simulink library "bpm_dq_S_noH_D_RL_U_HA_Spin_xk"  (R2022b)
settings: Solver=VariableStepAuto  StartTime=0.0  StopTime=10.0  RelTol=1e-3
Description:
  | Created by MapleSim.
settings Model: Creator=MapleSim  LastModifiedBy=BEDNASA

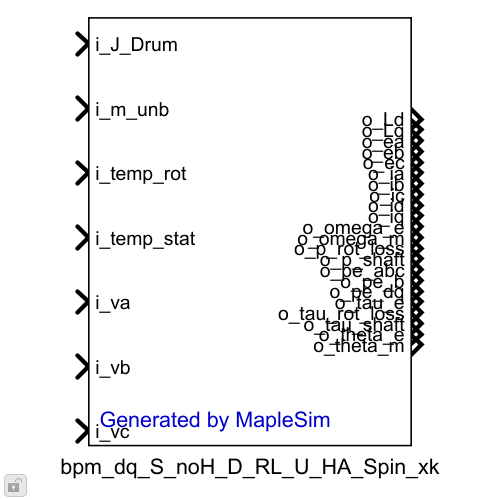
[thumbnail: Simulink's stored preview of the top-level diagram]
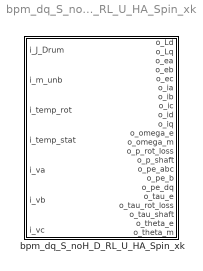
== system bpm_dq_S_noH_D_RL_U_HA_Spin_xk ==
  bpm_dq_S_noH_D_RL_U_HA_Spin_xk : Subsystem  Description=Subsystem: bpm_dq_S_noH_D_RL_U_HA_Spin_xk  mask(bpm_dq_S_noH_D_RL_U_HA_Spin_xk){ic=[0., 0., 0., -0., 0.], Par1=.1e-3, Par2=0., Par3=1., Par4=2., Par5=3., Par6=4., Par7=5., Par8=6., Par9=7., Par10=.515e-3, Par11=.884e-1, Par12=.2117e-1, Par13=.2117e-1, Par14=.2117e-1, Par15=.2117e-1, Par16=.2117e-1, Par17=.2117e-1, Par18=.2117e-1, Par19=.2117e-1, Par20=.972e-1, Par21=.2744e-1, Par22=.2777e-1, Par23=.2742e-1, Par24=.2646e-1, Par25=.2426e-1, Par26=.2329e-1, Par27=.2241e-1, Par28=.2241e-1, Par29=1., Par30=3., Par31=0., Par32=1., Par33=12., Par34=19., Par35=26., Par36=35., Par37=41., Par38=56., Par39=0., Par40=.5e3, Par41=.3e4, Par42=.4e4, Par43=.5e4, Par44=.7e4, Par45=.12e5, Par46=.18e5, Par47=1., Par48=.1e2, Par49=9.15, Par50=1., Par51=2., Par52=3., Par53=22., Par54=22., Par55=.2e-3, Par56=.4e-2, Par57=.206e-2, Par58=.1151, Par59=1., Par60=1., Par61=1., Par62=0., Par63=0., Par64=0., Par65=-9.8, Par66=-1., Par67=1., ExtData=, MinStep=1/40, TimeStep_Solver=1e-4}
      mask prompts: ic "Initial Conditions:"; Par1 "SHDRLUHAS1_B:"; Par2 "SHDRLUHAS1_I_pk0:"; Par3 "SHDRLUHAS1_I_pk1:"; Par4 "SHDRLUHAS1_I_pk2:"; Par5 "SHDRLUHAS1_I_pk3:"; Par6 "SHDRLUHAS1_I_pk4:"; Par7 "SHDRLUHAS1_I_pk5:"; Par8 "SHDRLUHAS1_I_pk6:"; Par9 "SHDRLUHAS1_I_pk7:"; Par10 "SHDRLUHAS1_Jrotor:"; Par11 "SHDRLUHAS1_Ld0:"; Par12 "SHDRLUHAS1_Ld_a0:"; Par13 "SHDRLUHAS1_Ld_a1:"; Par14 "SHDRLUHAS1_Ld_a2:"; Par15 "SHDRLUHAS1_Ld_a3:"; Par16 "SHDRLUHAS1_Ld_a4:"; Par17 "SHDRLUHAS1_Ld_a5:"; Par18 "SHDRLUHAS1_Ld_a6:"; Par19 "SHDRLUHAS1_Ld_a7:"; Par20 "SHDRLUHAS1_Lq0:"; Par21 "SHDRLUHAS1_Lq_b0:"; Par22 "SHDRLUHAS1_Lq_b1:"; Par23 "SHDRLUHAS1_Lq_b2:"; Par24 "SHDRLUHAS1_Lq_b3:"; Par25 "SHDRLUHAS1_Lq_b4:"; Par26 "SHDRLUHAS1_Lq_b5:"; Par27 "SHDRLUHAS1_Lq_b6:"; Par28 "SHDRLUHAS1_Lq_b7:"; Par29 "SHDRLUHAS1_Ls_Sat_enable:"; Par30 "SHDRLUHAS1_NPP:"; Par31 "SHDRLUHAS1_Rot_Loss_Power0:"; Par32 "SHDRLUHAS1_Rot_Loss_Power1:"; Par33 "SHDRLUHAS1_Rot_Loss_Power2:"; Par34 "SHDRLUHAS1_Rot_Loss_Power3:"; Par35 "SHDRLUHAS1_Rot_Loss_Power4:"; Par36 "SHDRLUHAS1_Rot_Loss_Power5:"; Par37 "SHDRLUHAS1_Rot_Loss_Power6:"; Par38 "SHDRLUHAS1_Rot_Loss_Power7:"; Par39 "SHDRLUHAS1_Rot_Loss_Speed0:"; Par40 "SHDRLUHAS1_Rot_Loss_Speed1:"; Par41 "SHDRLUHAS1_Rot_Loss_Speed2:"; Par42 "SHDRLUHAS1_Rot_Loss_Speed3:"; Par43 "SHDRLUHAS1_Rot_Loss_Speed4:"; Par44 "SHDRLUHAS1_Rot_Loss_Speed5:"; Par45 "SHDRLUHAS1_Rot_Loss_Speed6:"; Par46 "SHDRLUHAS1_Rot_Loss_Speed7:"; Par47 "SHDRLUHAS1_Rot_Loss_enable:"; Par48 "SHDRLUHAS1_Rot_Loss_omega_th:"; Par49 "SHDRLUHAS1_Rs0:"; Par50 "SHDRLUHAS1_Rsa_aux:"; Par51 "SHDRLUHAS1_Rsb_aux:"; Par52 "SHDRLUHAS1_Rsc_aux:"; Par53 "SHDRLUHAS1_TrRef:"; Par54 "SHDRLUHAS1_TsRef:"; Par55 "SHDRLUHAS1_Ts:"; Par56 "SHDRLUHAS1_alpha_s:"; Par57 "SHDRLUHAS1_d_magnet:"; Par58 "SHDRLUHAS1_phiPM1:"; Par59 "SHDRLUHAS1_HA_Spin_Mechanics_CF:"; Par60 "SHDRLUHAS1_HA_Spin_Mechanics_TR:"; Par61 "SHDRLUHAS1_HA_Spin_Mechanics_damp:"; Par62 "SHDRLUHAS1_HA_Spin_Mechanics_damper3_1_B:"; Par63 "SHDRLUHAS1_HA_Spin_Mechanics_damper3_1_C:"; Par64 "SHDRLUHAS1_HA_Spin_Mechanics_fixed_phi0:"; Par65 "SHDRLUHAS1_HA_Spin_Mechanics_gain11_k:"; Par66 "SHDRLUHAS1_HA_Spin_Mechanics_gain21_k:"; Par67 "SHDRLUHAS1_HA_Spin_Mechanics_r_unb:"; ExtData "Extended Visualization Data - File Name (leave blank to disable):"; MinStep "Extended Visualization Data - Minimum Sample Step:"; TimeStep_Solver "Time Step - Solver:"
      mask help:
      | Variable Definitions
      |
      | Variable(s) in the Initial Condition Vector:
      |      x[ 0] = `Main.SHDRLUHAS1.o_id`(t)
      |      x[ 1] = `Main.SHDRLUHAS1.o_iq`(t)
      |      x[ 2] = `Main.SHDRLUHAS1.o_omega_e`(t)
      |      x[ 3] = `Main.SHDRLUHAS1.o_theta_e`(t)
      |      x[ 4] = diff(`Main.SHDRLUHAS1.o_theta_e`(t),t)
      |
      | Variable(s) in the Output Vector:
      |    o_Ld:
      |      y[ 0] = `Main.SHDRLUHAS1.o_Ld`(t)
      |    o_Lq:
      |      y[ 1] = `Main.SHDRLUHAS1.o_Lq`(t)
      |    o_ea:
      |      y[ 2] = `Main.SHDRLUHAS1.o_ea`(t)
      |    o_eb:
      |      y[ 3] = `Main.SHDRLUHAS1.o_eb`(t)
      |    o_ec:
      |      y[ 4] = `Main.SHDRLUHAS1.o_ec`(t)
      |    o_ia:
      |      y[ 5] = `Main.SHDRLUHAS1.o_ia`(t)
      |    o_ib:
      |      y[ 6] = `Main.SHDRLUHAS1.o_ib`(t)
      |    o_ic:
      |      y[ 7] = `Main.SHDRLUHAS1.o_ic`(t)
      |    o_id:
      |      y[ 8] = `Main.SHDRLUHAS1.o_id`(t)
      |    o_iq:
      |      y[ 9] = `Main.SHDRLUHAS1.o_iq`(t)
      |    o_omega_e:
      |      y[10] = `Main.SHDRLUHAS1.o_omega_e`(t)
      |    o_omega_m:
      |      y[11] = `Main.SHDRLUHAS1.o_omega_m`(t)
      |    o_p_rot_loss:
      |      y[12] = `Main.SHDRLUHAS1.o_p_rot_loss`(t)
      |    o_p_shaft:
      |      y[13] = `Main.SHDRLUHAS1.o_p_shaft`(t)
      |    o_pe_abc:
      |      y[14] = `Main.SHDRLUHAS1.o_pe_abc`(t)
      |    o_pe_b:
      |      y[15] = `Main.SHDRLUHAS1.o_pe_b`(t)
      |    o_pe_dq:
      |      y[16] = `Main.SHDRLUHAS1.o_pe_dq`(t)
      |    o_tau_e:
      |      y[17] = `Main.SHDRLUHAS1.o_tau_e`(t)
      |    o_tau_rot_loss:
      |      y[18] = `Main.SHDRLUHAS1.o_tau_rot_loss`(t)
      |    o_tau_shaft:
      |      y[19] = `Main.SHDRLUHAS1.o_tau_shaft`(t)
      |    o_theta_e:
      |      y[20] = `Main.SHDRLUHAS1.o_theta_e`(t)
      |    o_theta_m:
      |      y[21] = `Main.SHDRLUHAS1.o_theta_m`(t)
      |
      | Variable(s) in the Input Vector:
      |    i_J_Drum:
      |      y[ 0] = `Main.SHDRLUHAS1.i_J_Drum`(t)
      |    i_m_unb:
      |      y[ 1] = `Main.SHDRLUHAS1.i_m_unb`(t)
      |    i_temp_rot:
      |      y[ 2] = `Main.SHDRLUHAS1.i_temp_rot`(t)
      |    i_temp_stat:
      |      y[ 3] = `Main.SHDRLUHAS1.i_temp_stat`(t)
      |    i_va:
      |      y[ 4] = `Main.SHDRLUHAS1.i_va`(t)
      |    i_vb:
      |      y[ 5] = `Main.SHDRLUHAS1.i_vb`(t)
      |    i_vc:
      |      y[ 6] = `Main.SHDRLUHAS1.i_vc`(t)
      |
      | Parameter(s):
      |      p[ 0] = `Main.SHDRLUHAS1.B` (default = .1e-3)
      |      p[ 1] = `Main.SHDRLUHAS1.I_pk0` (default = 0.)
      |      p[ 2] = `Main.SHDRLUHAS1.I_pk1` (default = 1.)
      |      p[ 3] = `Main.SHDRLUHAS1.I_pk2` (default = 2.)
      |      p[ 4] = `Main.SHDRLUHAS1.I_pk3` (default = 3.)
      |      p[ 5] = `Main.SHDRLUHAS1.I_pk4` (default = 4.)
      |      p[ 6] = `Main.SHDRLUHAS1.I_pk5` (default = 5.)
      |      p[ 7] = `Main.SHDRLUHAS1.I_pk6` (default = 6.)
      |      p[ 8] = `Main.SHDRLUHAS1.I_pk7` (default = 7.)
      |      p[ 9] = `Main.SHDRLUHAS1.Jrotor` (default = .515e-3)
      |      p[10] = `Main.SHDRLUHAS1.Ld0` (default = .884e-1)
      |      p[11] = `Main.SHDRLUHAS1.Ld_a0` (default = .2117e-1)
      |      p[12] = `Main.SHDRLUHAS1.Ld_a1` (default = .2117e-1)
      |      p[13] = `Main.SHDRLUHAS1.Ld_a2` (default = .2117e-1)
      |      p[14] = `Main.SHDRLUHAS1.Ld_a3` (default = .2117e-1)
      |      p[15] = `Main.SHDRLUHAS1.Ld_a4` (default = .2117e-1)
      |      p[16] = `Main.SHDRLUHAS1.Ld_a5` (default = .2117e-1)
      |      p[17] = `Main.SHDRLUHAS1.Ld_a6` (default = .2117e-1)
      |      p[18] = `Main.SHDRLUHAS1.Ld_a7` (default = .2117e-1)
      |      p[19] = `Main.SHDRLUHAS1.Lq0` (default = .972e-1)
      |      p[20] = `Main.SHDRLUHAS1.Lq_b0` (default = .2744e-1)
      |      p[21] = `Main.SHDRLUHAS1.Lq_b1` (default = .2777e-1)
      |      p[22] = `Main.SHDRLUHAS1.Lq_b2` (default = .2742e-1)
      |      p[23] = `Main.SHDRLUHAS1.Lq_b3` (default = .2646e-1)
      |      p[24] = `Main.SHDRLUHAS1.Lq_b4` (default = .2426e-1)
      |      p[25] = `Main.SHDRLUHAS1.Lq_b5` (default = .2329e-1)
      |      p[26] = `Main.SHDRLUHAS1.Lq_b6` (default = .2241e-1)
      |      p[27] = `Main.SHDRLUHAS1.Lq_b7` (default = .2241e-1)
      |      p[28] = `Main.SHDRLUHAS1.Ls_Sat_enable` (default = 1.)
      |      p[29] = `Main.SHDRLUHAS1.NPP` (default = 3.)
      |      p[30] = `Main.SHDRLUHAS1.Rot_Loss_Power0` (default = 0.)
      |      p[31] = `Main.SHDRLUHAS1.Rot_Loss_Power1` (default = 1.)
      |      p[32] = `Main.SHDRLUHAS1.Rot_Loss_Power2` (default = 12.)
      |      p[33] = `Main.SHDRLUHAS1.Rot_Loss_Power3` (default = 19.)
      |      p[34] = `Main.SHDRLUHAS1.Rot_Loss_Power4` (default = 26.)
      |      p[35] = `Main.SHDRLUHAS1.Rot_Loss_Power5` (default = 35.)
      |      p[36] = `Main.SHDRLUHAS1.Rot_Loss_Power6` (default = 41.)
      |      p[37] = `Main.SHDRLUHAS1.Rot_Loss_Power7` (default = 56.)
      |      p[38] = `Main.SHDRLUHAS1.Rot_Loss_Speed0` (default = 0.)
      |      p[39] = `Main.SHDRLUHAS1.Rot_Loss_Speed1` (default = .5e3)
      |      p[40] = `Main.SHDRLUHAS1.Rot_Loss_Speed2` (default = .3e4)
      |      p[41] = `Main.SHDRLUHAS1.Rot_Loss_Speed3` (default = .4e4)
      |      p[42] = `Main.SHDRLUHAS1.Rot_Loss_Speed4` (default = .5e4)
      |      p[43] = `Main.SHDRLUHAS1.Rot_Loss_Speed5` (default = .7e4)
      |      p[44] = `Main.SHDRLUHAS1.Rot_Loss_Speed6` (default = .12e5)
      |      p[45] = `Main.SHDRLUHAS1.Rot_Loss_Speed7` (default = .18e5)
      |      p[46] = `Main.SHDRLUHAS1.Rot_Loss_enable` (default = 1.)
      |      p[47] = `Main.SHDRLUHAS1.Rot_Loss_omega_th` (default = .1e2)
      |      p[48] = `Main.SHDRLUHAS1.Rs0` (default = 9.15)
      |      p[49] = `Main.SHDRLUHAS1.Rsa_aux` (default = 1.)
      |      p[50] = `Main.SHDRLUHAS1.Rsb_aux` (default = 2.)
      |      p[51] = `Main.SHDRLUHAS1.Rsc_aux` (default = 3.)
      |      p[52] = `Main.SHDRLUHAS1.TrRef` (default = 22.)
      |      p[53] = `Main.SHDRLUHAS1.TsRef` (default = 22.)
      |      p[54] = `Main.SHDRLUHAS1.Ts` (default = .2e-3)
      |      p[55] = `Main.SHDRLUHAS1.alpha_s` (default = .4e-2)
      |      p[56] = `Main.SHDRLUHAS1.d_magnet` (default = .206e-2)
      |      p[57] = `Main.SHDRLUHAS1.phiPM1` (default = .1151)
      |      p[58] = `Main.SHDRLUHAS1.HA_Spin_Mechanics.CF` (default = 1.)
      |      p[59] = `Main.SHDRLUHAS1.HA_Spin_Mechanics.TR` (default = 1.)
      |      p[60] = `Main.SHDRLUHAS1.HA_Spin_Mechanics.damp` (default = 1.)
      |      p[61] = `Main.SHDRLUHAS1.HA_Spin_Mechanics.damper3_1.B` (default = 0.)
      |      p[62] = `Main.SHDRLUHAS1.HA_Spin_Mechanics.damper3_1.C` (default = 0.)
      |      p[63] = `Main.SHDRLUHAS1.HA_Spin_Mechanics.fixed.phi0` (default = 0.)
      |      p[64] = `Main.SHDRLUHAS1.HA_Spin_Mechanics.gain11.k` (default = -9.8)
      |      p[65] = `Main.SHDRLUHAS1.HA_Spin_Mechanics.gain21.k` (default = -1.)
      |      p[66] = `Main.SHDRLUHAS1.HA_Spin_Mechanics.r_unb` (default = 1.)
      mask Help: <!DOCTYPE html PUBLIC "-//W3C//DTD HTML 4.01 Transitional//EN" "http://www.w3.org/TR/1999/REC-html401-19991224/loose.dtd"> <html lang="en"> <head> <title>bpm_dq_S_noH_D_RL_U_HA_Spin_xk :: MapleSim model</title> <style type="text/css"> body { background-color: white; margin:10px;} h1 { color: #990000; font-size: x-large; } h2 { color: #990000; font-size: large; margin-top:0ex;     margin-bottom:0ex;   font-weight:bold;  } h3 { color:#990000;  margin-top:0ex;   margin-bottom:0ex;  font-weight:bold;    font-size: medium; } h4 { color:black;    margin-top:0ex;   margin-bottom:0ex;  font-weight:bold;    font-size: medium; } /* Vertical space in tables other than the header and footer banners */ table.body { margin-top: 2ex; margin-bottom: 2ex;} /* Make the text shrink to fit narrow windows, but not stretch too far in wide windows. */ p,h1,h2,div.content div { max-width: 600px; } pre.codeinput { background: #EEEEEE; padding: 10px;} @media print { pre.codeinput { word-wrap:break-word; width:100%; } } span.keyword { color: #0000FF} span.comment { color: #228B22} span.string { color: #A020F0} span.untermstring {color: #B20000} span.syscmd { color: #B28C00} pre.error { color: red;} p.footer { text-align: right; font-size: xx-small; font-weight: lighter; font-style: italic; color: gray; } </style> <meta name="generator" content="DocBook XSL Stylesheets V1.52.2"> <meta name="chunktype" content="refpage"> <meta http-equiv="Content-Script-Type" content="text/javascript"> </head> <body> <a name="top_of_page"></a> <p style="font-size:1px;"> <a name="f8-894621"></a> <a name="transferfcn"></a> <a class="indexterm" name="zmw57dd0e42758"></a></p> <h1 class="reftitle">bpm_dq_S_noH_D_RL_U_HA_Spin_xk</h1> <p>Simulink Block generated by MapleSim Connector</p> <p><a name="f8-894627"></a></p> <h1>Description <span class="inlinemediaobject"></span></h1> <p><a class="indexterm" name="zmw57dd0e42781"></a></p> <p>The bpm_dq_S_noH_D_RL_U_HA_Spin_xk model runs in the continuous domain and is created in the MapleSim modeling environment. The discrete S-Function block bpm_dq_S_noH_D_RL_U_HA_Spin_xk is created using MapleSim Connector. The block is a 7-input, 22-output, 67-parameter system.</p> <p><a name="f8-894641"></a></p> <h1>System Variables</h1> <p>The following variables are used in the S-Function block:</p>  State Variable(s)<dl><dd>x[ 0] = `Main.SHDRLUHAS1.o_id`(t)</dd></br><dd>x[ 1] = `Main.SHDRLUHAS1.o_iq`(t)</dd></br><dd>x[ 2] = `Main.SHDRLUHAS1.o_omega_e`(t)</dd></br><dd>x[ 3] = `Main.SHDRLUHAS1.o_theta_e`(t)</dd></br><dd>x[ 4] = diff(`Main.SHDRLUHAS1.o_theta_e`(t),t)</dd></br></dl> Output Variable(s)<dl><dd>o_Ld:</dd></br><dd>&nbsp;&nbsp;y[ 0] = `Main.SHDRLUHAS1.o_Ld`(t)</dd></br><dd>o_Lq:</dd></br><dd>&nbsp;&nbsp;y[ 1] = `Main.SHDRLUHAS1.o_Lq`(t)</dd></br><dd>o_ea:</dd></br><dd>&nbsp;&nbsp;y[ 2] = `Main.SHDRLUHAS1.o_ea`(t)</dd></br><dd>o_eb:</dd></br><dd>&nbsp;&nbsp;y[ 3] = `Main.SHDRLUHAS1.o_eb`(t)</dd></br><dd>o_ec:</dd></br><dd>&nbsp;&nbsp;y[ 4] = `Main.SHDRLUHAS1.o_ec`(t)</dd></br><dd>o_ia:</dd></br><dd>&nbsp;&nbsp;y[ 5] = `Main.SHDRLUHAS1.o_ia`(t)</dd></br><dd>o_ib:</dd></br><dd>&nbsp;&nbsp;y[ 6] = `Main.SHDRLUHAS1.o_ib`(t)</dd></br><dd>o_ic:</dd></br><dd>&nbsp;&nbsp;y[ 7] = `Main.SHDRLUHAS1.o_ic`(t)</dd></br><dd>o_id:</dd></br><dd>&nbsp;&nbsp;y[ 8] = `Main.SHDRLUHAS1.o_id`(t)</dd></br><dd>o_iq:</dd></br><dd>&nbsp;&nbsp;y[ 9] = `Main.SHDRLUHAS1.o_iq`(t)</dd></br><dd>o_omega_e:</dd></br><dd>&nbsp;&nbsp;y[10] = `Main.SHDRLUHAS1.o_omega_e`(t)</dd></br><dd>o_omega_m:</dd></br><dd>&nbsp;&nbsp;y[11] = `Main.SHDRLUHAS1.o_omega_m`(t)</dd></br><dd>o_p_rot_loss:</dd></br><dd>&nbsp;&nbsp;y[12] = `Main.SHDRLUHAS1.o_p_rot_loss`(t)</dd></br><dd>o_p_shaft:</dd></br><dd>&nbsp;&nbsp;y[13] = `Main.SHDRLUHAS1.o_p_shaft`(t)</dd></br><dd>o_pe_abc:</dd></br><dd>&nbsp;&nbsp;y[14] = `Main.SHDRLUHAS1.o_pe_abc`(t)</dd></br><dd>o_pe_b:</dd></br><dd>&nbsp;&nbsp;y[15] = `Main.SHDRLUHAS1.o_pe_b`(t)</dd></br><dd>o_pe_dq:</dd></br><dd>&nbsp;&nbsp;y[16] = `Main.SHDRLUHAS1.o_pe_dq`(t)</dd></br><dd>o_tau_e:</dd></br><dd>&nbsp;&nbsp;y[17] = `Main.SHDRLUHAS1.o_tau_e`(t)</dd></br><dd>o_tau_rot_loss:</dd></br><dd>&nbsp;&nbsp;y[18] = `Main.SHDRLUHAS1.o_tau_rot_loss`(t)</dd></br><dd>o_tau_shaft:</dd></br><dd>&nbsp;&nbsp;y[19] = `Main.SHDRLUHAS1.o_tau_shaft`(t)</dd></br><dd>o_theta_e:</dd></br><dd>&nbsp;&nbsp;y[20] = `Main.SHDRLUHAS1.o_theta_e`(t)</dd></br><dd>o_theta_m:</dd></br><dd>&nbsp;&nbsp;y[21] = `Main.SHDRLUHAS1.o_theta_m`(t)</dd></br></dl> Input Variable(s)<dl><dd>i_J_Drum:</dd></br><dd>&nbsp;&nbsp;y[ 0] = `Main.SHDRLUHAS1.i_J_Drum`(t)</dd></br><dd>i_m_unb:</dd></br><dd>&nbsp;&nbsp;y[ 1] = `Main.SHDRLUHAS1.i_m_unb`(t)</dd></br><dd>i_temp_rot:</dd></br><dd>&nbsp;&nbsp;y[ 2] = `Main.SHDRLUHAS1.i_temp_rot`(t)</dd></br><dd>i_temp_stat:</dd></br><dd>&nbsp;&nbsp;y[ 3] = `Main.SHDRLUHAS1.i_temp_stat`(t)</dd></br><dd>i_va:</dd></br><dd>&nbsp;&nbsp;y[ 4] = `Main.SHDRLUHAS1.i_va`(t)</dd></br><dd>i_vb:</dd></br><dd>&nbsp;&nbsp;y[ 5] = `Main.SHDRLUHAS1.i_vb`(t)</dd></br><dd>i_vc:</dd></br><dd>&nbsp;&nbsp;y[ 6] = `Main.SHDRLUHAS1.i_vc`(t)</dd></br></dl> Parameter(s)<dl><dd>p[ 0] = `Main.SHDRLUHAS1.B` (default = .1e-3)</dd></br><dd>p[ 1] = `Main.SHDRLUHAS1.I_pk0` (default = 0.)</dd></br><dd>p[ 2] = `Main.SHDRLUHAS1.I_pk1` (default = 1.)</dd></br><dd>p[ 3] = `Main.SHDRLUHAS1.I_pk2` (default = 2.)</dd></br><dd>p[ 4] = `Main.SHDRLUHAS1.I_pk3` (default = 3.)</dd></br><dd>p[ 5] = `Main.SHDRLUHAS1.I_pk4` (default = 4.)</dd></br><dd>p[ 6] = `Main.SHDRLUHAS1.I_pk5` (default = 5.)</dd></br><dd>p[ 7] = `Main.SHDRLUHAS1.I_pk6` (default = 6.)</dd></br><dd>p[ 8] = `Main.SHDRLUHAS1.I_pk7` (default = 7.)</dd></br><dd>p[ 9] = `Main.SHDRLUHAS1.Jrotor` (default = .515e-3)</dd></br><dd>p[10] = `Main.SHDRLUHAS1.Ld0` (default = .884e-1)</dd></br><dd>p[11] = `Main.SHDRLUHAS1.Ld_a0` (default = .2117e-1)</dd></br><dd>p[12] = `Main.SHDRLUHAS1.Ld_a1` (default = .2117e-1)</dd></br><dd>p[13] = `Main.SHDRLUHAS1.Ld_a2` (default = .2117e-1)</dd></br><dd>p[14] = `Main.SHDRLUHAS1.Ld_a3` (default = .2117e-1)</dd></br><dd>p[15] = `Main.SHDRLUHAS1.Ld_a4` (default = .2117e-1)</dd></br><dd>p[16] = `Main.SHDRLUHAS1.Ld_a5` (default = .2117e-1)</dd></br><dd>p[17] = `Main.SHDRLUHAS1.Ld_a6` (default = .2117e-1)</dd></br><dd>p[18] = `Main.SHDRLUHAS1.Ld_a7` (default = .2117e-1)</dd></br><dd>p[19] = `Main.SHDRLUHAS1.Lq0` (default = .972e-1)</dd></br><dd>p[20] = `Main.SHDRLUHAS1.Lq_b0` (default = .2744e-1)</dd></br><dd>p[21] = `Main.SHDRLUHAS1.Lq_b1` (default = .2777e-1)</dd></br><dd>p[22] = `Main.SHDRLUHAS1.Lq_b2` (default = .2742e-1)</dd></br><dd>p[23] = `Main.SHDRLUHAS1.Lq_b3` (default = .2646e-1)</dd></br><dd>p[24] = `Main.SHDRLUHAS1.Lq_b4` (default = .2426e-1)</dd></br><dd>p[25] = `Main.SHDRLUHAS1.Lq_b5` (default = .2329e-1)</dd></br><dd>p[26] = `Main.SHDRLUHAS1.Lq_b6` (default = .2241e-1)</dd></br><dd>p[27] = `Main.SHDRLUHAS1.Lq_b7` (default = .2241e-1)</dd></br><dd>p[28] = `Main.SHDRLUHAS1.Ls_Sat_enable` (default = 1.)</dd></br><dd>p[29] = `Main.SHDRLUHAS1.NPP` (default = 3.)</dd></br><dd>p[30] = `Main.SHDRLUHAS1.Rot_Loss_Power0` (default = 0.)</dd></br><dd>p[31] = `Main.SHDRLUHAS1.Rot_Loss_Power1` (default = 1.)</dd></br><dd>p[32] = `Main.SHDRLUHAS1.Rot_Loss_Power2` (default = 12.)</dd></br><dd>p[33] = `Main.SHDRLUHAS1.Rot_Loss_Power3` (default = 19.)</dd></br><dd>p[34] = `Main.SHDRLUHAS1.Rot_Loss_Power4` (default = 26.)</dd></br><dd>p[35] = `Main.SHDRLUHAS1.Rot_Loss_Power5` (default = 35.)</dd></br><dd>p[36] = `Main.SHDRLUHAS1.Rot_Loss_Power6` (default = 41.)</dd></br><dd>p[37] = `Main.SHDRLUHAS1.Rot_Loss_Power7` (default = 56.)</dd></br><dd>p[38] = `Main.SHDRLUHAS1.Rot_Loss_Speed0` (default = 0.)</dd></br><dd>p[39] = `Main.SHDRLUHAS1.Rot_Loss_Speed1` (default = .5e3)</dd></br><dd>p[40] = `Main.SHDRLUHAS1.Rot_Loss_Speed2` (default = .3e4)</dd></br><dd>p[41] = `Main.SHDRLUHAS1.Rot_Loss_Speed3` (default = .4e4)</dd></br><dd>p[42] = `Main.SHDRLUHAS1.Rot_Loss_Speed4` (default = .5e4)</dd></br><dd>p[43] = `Main.SHDRLUHAS1.Rot_Loss_Speed5` (default = .7e4)</dd></br><dd>p[44] = `Main.SHDRLUHAS1.Rot_Loss_Speed6` (default = .12e5)</dd></br><dd>p[45] = `Main.SHDRLUHAS1.Rot_Loss_Speed7` (default = .18e5)</dd></br><dd>p[46] = `Main.SHDRLUHAS1.Rot_Loss_enable` (default = 1.)</dd></br><dd>p[47] = `Main.SHDRLUHAS1.Rot_Loss_omega_th` (default = .1e2)</dd></br><dd>p[48] = `Main.SHDRLUHAS1.Rs0` (default = 9.15)</dd></br><dd>p[49] = `Main.SHDRLUHAS1.Rsa_aux` (default = 1.)</dd></br><dd>p[50] = `Main.SHDRLUHAS1.Rsb_aux` (default = 2.)</dd></br><dd>p[51] = `Main.SHDRLUHAS1.Rsc_aux` (default = 3.)</dd></br><dd>p[52] = `Main.SHDRLUHAS1.TrRef` (default = 22.)</dd></br><dd>p[53] = `Main.SHDRLUHAS1.TsRef` (default = 22.)</dd></br><dd>p[54] = `Main.SHDRLUHAS1.Ts` (default = .2e-3)</dd></br><dd>p[55] = `Main.SHDRLUHAS1.alpha_s` (default = .4e-2)</dd></br><dd>p[56] = `Main.SHDRLUHAS1.d_magnet` (default = .206e-2)</dd></br><dd>p[57] = `Main.SHDRLUHAS1.phiPM1` (default = .1151)</dd></br><dd>p[58] = `Main.SHDRLUHAS1.HA_Spin_Mechanics.CF` (default = 1.)</dd></br><dd>p[59] = `Main.SHDRLUHAS1.HA_Spin_Mechanics.TR` (default = 1.)</dd></br><dd>p[60] = `Main.SHDRLUHAS1.HA_Spin_Mechanics.damp` (default = 1.)</dd></br><dd>p[61] = `Main.SHDRLUHAS1.HA_Spin_Mechanics.damper3_1.B` (default = 0.)</dd></br><dd>p[62] = `Main.SHDRLUHAS1.HA_Spin_Mechanics.damper3_1.C` (default = 0.)</dd></br><dd>p[63] = `Main.SHDRLUHAS1.HA_Spin_Mechanics.fixed.phi0` (default = 0.)</dd></br><dd>p[64] = `Main.SHDRLUHAS1.HA_Spin_Mechanics.gain11.k` (default = -9.8)</dd></br><dd>p[65] = `Main.SHDRLUHAS1.HA_Spin_Mechanics.gain21.k` (default = -1.)</dd></br><dd>p[66] = `Main.SHDRLUHAS1.HA_Spin_Mechanics.r_unb` (default = 1.)</dd></br></dl></p> <p><a name="f8-894651"></a></p><h1>Data Type Support</h1> <p>The bpm_dq_S_noH_D_RL_U_HA_Spin_xk block accepts inputs and outputs signals of type <tt>double</tt>.</p> <a name="f8-894653"></a><h1>Parameters</h1><dl> <dt><a name="zmw57dd0e42948"></a><b><span class="term">Initial Condition</span>s</b></dt> <dd> <p>The row vector of initial conditions. A vector can be specified to initialize the state variables of the system.</p></dd> <dt><a name="zmw57dd0e42958"></a><span class="term"><b>Parameters</b></span></dt> <dd> <p>The scalars or the row vector of tunable parameters.</p></dd> </dl> <dt><a name="zmw57dd0e42968"></a> </dt><h1>Characteristics</h1> <table cellspacing="0" class="body" cellpadding="4" border="2"><colgroup><col width="41%"><col width="59%"></colgroup><tbody> <tr valign="top"><td bgcolor="#F2F2F2"><p>Direct Feedthrough</p></td><td bgcolor="#F2F2F2"><p>Yes, only if the block has no state variables.</p></td></tr> <tr valign="top"><td bgcolor="#F2F2F2"><p>Sample Time</p></td><td bgcolor="#F2F2F2"><p> Discrete</p></td></tr> <tr valign="top"><td bgcolor="#F2F2F2"><p>Scalar Expansion</p></td><td bgcolor="#F2F2F2"><p>No</p></td></tr> <tr valign="top"><td bgcolor="#F2F2F2"><p>State</p></td><td bgcolor="#F2F2F2"><p>Yes</p></td></tr> <tr valign="top"><td bgcolor="#F2F2F2"><p>Dimensionalized</p></td><td bgcolor="#F2F2F2"><p>Yes</p></td></tr> <tr valign="top"><td bgcolor="#F2F2F2"><p>Zero Crossing</p></td><td bgcolor="#F2F2F2"><p>Yes</p></td></tr> </tbody></table> <p></p><h1>Maple / MapleSim / MapleSim Connector Details</h1> <p></p><dd><p>Maple 2021.1, X86 64 WINDOWS, May 19 2021, Build ID 1539851</p></dd><dd><p>MapleSim 2021.1 Control Design, Wed May 19 23:38:09 EDT 2021, 1539851</p></dd><dd><p>MapleSim 2021.1 Connector for FMI, Wed May 19 23:38:47 EDT 2021, 1539851</p></dd><dd><p>GlobalOptimization 2021.0, Thu Mar 11 13:21:11 EST 2021, 1524228</p></dd><dd><p>MapleSim 2021.1, Wed May 19 23:37:53 EDT 2021, 1539851</p></dd><dd><p>MapleSim 2021.1 Connector, Wed May 19 23:39:01 EDT 2021, 1539851</p></dd><p></p></body></html>
      mask Display: color('blue');text(5,12,'Generated by MapleSim');

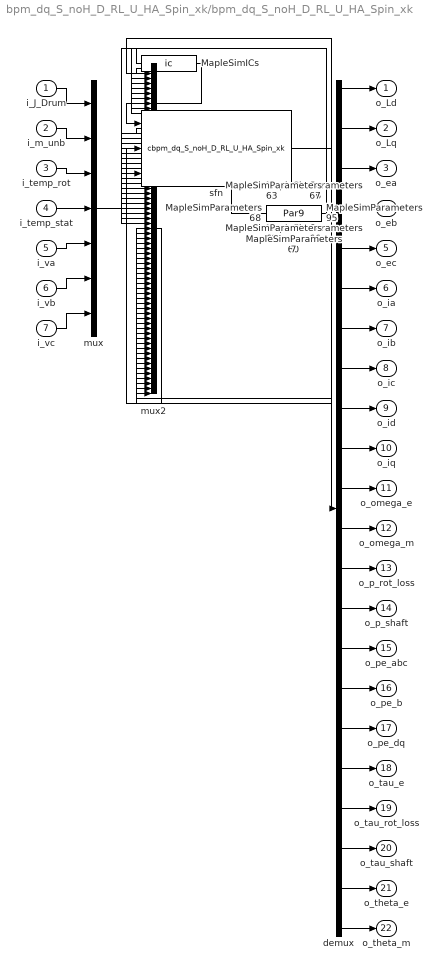
== system bpm_dq_S_noH_D_RL_U_HA_Spin_xk/bpm_dq_S_noH_D_RL_U_HA_Spin_xk ==
  i_J_Drum : Inport
  i_m_unb : Inport  Port=2
  i_temp_rot : Inport  Port=3
  i_temp_stat : Inport  Port=4
  i_va : Inport  Port=5
  i_vb : Inport  Port=6
  i_vc : Inport  Port=7
  MapleSimICs : Constant  Value=ic
  MapleSimParameters1 : Constant  Value=Par1
  MapleSimParameters10 : Constant  Value=Par10
  MapleSimParameters11 : Constant  Value=Par11
  MapleSimParameters12 : Constant  Value=Par12
  MapleSimParameters13 : Constant  Value=Par13
  MapleSimParameters14 : Constant  Value=Par14
  MapleSimParameters15 : Constant  Value=Par15
  MapleSimParameters16 : Constant  Value=Par16
  MapleSimParameters17 : Constant  Value=Par17
  MapleSimParameters18 : Constant  Value=Par18
  MapleSimParameters19 : Constant  Value=Par19
  MapleSimParameters2 : Constant  Value=Par2
  MapleSimParameters20 : Constant  Value=Par20
  MapleSimParameters21 : Constant  Value=Par21
  MapleSimParameters22 : Constant  Value=Par22
  MapleSimParameters23 : Constant  Value=Par23
  MapleSimParameters24 : Constant  Value=Par24
  MapleSimParameters25 : Constant  Value=Par25
  MapleSimParameters26 : Constant  Value=Par26
  MapleSimParameters27 : Constant  Value=Par27
  MapleSimParameters28 : Constant  Value=Par28
  MapleSimParameters29 : Constant  Value=Par29
  MapleSimParameters3 : Constant  Value=Par3
  MapleSimParameters30 : Constant  Value=Par30
  MapleSimParameters31 : Constant  Value=Par31
  MapleSimParameters32 : Constant  Value=Par32
  MapleSimParameters33 : Constant  Value=Par33
  MapleSimParameters34 : Constant  Value=Par34
  MapleSimParameters35 : Constant  Value=Par35
  MapleSimParameters36 : Constant  Value=Par36
  MapleSimParameters37 : Constant  Value=Par37
  MapleSimParameters38 : Constant  Value=Par38
  MapleSimParameters39 : Constant  Value=Par39
  MapleSimParameters4 : Constant  Value=Par4
  MapleSimParameters40 : Constant  Value=Par40
  MapleSimParameters41 : Constant  Value=Par41
  MapleSimParameters42 : Constant  Value=Par42
  MapleSimParameters43 : Constant  Value=Par43
  MapleSimParameters44 : Constant  Value=Par44
  MapleSimParameters45 : Constant  Value=Par45
  MapleSimParameters46 : Constant  Value=Par46
  MapleSimParameters47 : Constant  Value=Par47
  MapleSimParameters48 : Constant  Value=Par48
  MapleSimParameters49 : Constant  Value=Par49
  MapleSimParameters5 : Constant  Value=Par5
  MapleSimParameters50 : Constant  Value=Par50
  MapleSimParameters51 : Constant  Value=Par51
  MapleSimParameters52 : Constant  Value=Par52
  MapleSimParameters53 : Constant  Value=Par53
  MapleSimParameters54 : Constant  Value=Par54
  MapleSimParameters55 : Constant  Value=Par55
  MapleSimParameters56 : Constant  Value=Par56
  MapleSimParameters57 : Constant  Value=Par57
  MapleSimParameters58 : Constant  Value=Par58
  MapleSimParameters59 : Constant  Value=Par59
  MapleSimParameters6 : Constant  Value=Par6
  MapleSimParameters60 : Constant  Value=Par60
  MapleSimParameters61 : Constant  Value=Par61
  MapleSimParameters62 : Constant  Value=Par62
  MapleSimParameters63 : Constant  Value=Par63
  MapleSimParameters64 : Constant  Value=Par64
  MapleSimParameters65 : Constant  Value=Par65
  MapleSimParameters66 : Constant  Value=Par66
  MapleSimParameters67 : Constant  Value=Par67
  MapleSimParameters7 : Constant  Value=Par7
  MapleSimParameters8 : Constant  Value=Par8
  MapleSimParameters9 : Constant  Value=Par9
  demux : Demux  Outputs=[1 1 1 1 1 1 1 1 1 1 1 1 1 1 1 1 1 1 1 1 1 1]
  mux : Mux  Inputs=7
  mux2 : Mux  Inputs=67
  sfn : S-Function  Description=Generated by MapleSim  FunctionName=cbpm_dq_S_noH_D_RL_U_HA_Spin_xk  Parameters=ExtData,MinStep,TimeStep_Solver  PortCounts=[3, 1]  SFunctionDeploymentMode=off  EnableBusSupport=off
  o_Ld : Outport
  o_Lq : Outport  Port=2
  o_ea : Outport  Port=3
  o_eb : Outport  Port=4
  o_ec : Outport  Port=5
  o_ia : Outport  Port=6
  o_ib : Outport  Port=7
  o_ic : Outport  Port=8
  o_id : Outport  Port=9
  o_iq : Outport  Port=10
  o_omega_e : Outport  Port=11
  o_omega_m : Outport  Port=12
  o_p_rot_loss : Outport  Port=13
  o_p_shaft : Outport  Port=14
  o_pe_abc : Outport  Port=15
  o_pe_b : Outport  Port=16
  o_pe_dq : Outport  Port=17
  o_tau_e : Outport  Port=18
  o_tau_rot_loss : Outport  Port=19
  o_tau_shaft : Outport  Port=20
  o_theta_e : Outport  Port=21
  o_theta_m : Outport  Port=22
  wires:
  MapleSimICs/1 -> sfn/1
  MapleSimParameters1/1 -> mux2/1
  MapleSimParameters2/1 -> mux2/2
  MapleSimParameters3/1 -> mux2/3
  MapleSimParameters4/1 -> mux2/4
  MapleSimParameters5/1 -> mux2/5
  MapleSimParameters6/1 -> mux2/6
  MapleSimParameters7/1 -> mux2/7
  MapleSimParameters8/1 -> mux2/8
  MapleSimParameters9/1 -> mux2/9
  MapleSimParameters10/1 -> mux2/10
  MapleSimParameters11/1 -> mux2/11
  MapleSimParameters12/1 -> mux2/12
  MapleSimParameters13/1 -> mux2/13
  MapleSimParameters14/1 -> mux2/14
  MapleSimParameters15/1 -> mux2/15
  MapleSimParameters16/1 -> mux2/16
  MapleSimParameters17/1 -> mux2/17
  MapleSimParameters18/1 -> mux2/18
  MapleSimParameters19/1 -> mux2/19
  MapleSimParameters20/1 -> mux2/20
  MapleSimParameters21/1 -> mux2/21
  MapleSimParameters22/1 -> mux2/22
  MapleSimParameters23/1 -> mux2/23
  MapleSimParameters24/1 -> mux2/24
  MapleSimParameters25/1 -> mux2/25
  MapleSimParameters26/1 -> mux2/26
  MapleSimParameters27/1 -> mux2/27
  MapleSimParameters28/1 -> mux2/28
  MapleSimParameters29/1 -> mux2/29
  MapleSimParameters30/1 -> mux2/30
  MapleSimParameters31/1 -> mux2/31
  MapleSimParameters32/1 -> mux2/32
  MapleSimParameters33/1 -> mux2/33
  MapleSimParameters34/1 -> mux2/34
  MapleSimParameters35/1 -> mux2/35
  MapleSimParameters36/1 -> mux2/36
  MapleSimParameters37/1 -> mux2/37
  MapleSimParameters38/1 -> mux2/38
  MapleSimParameters39/1 -> mux2/39
  MapleSimParameters40/1 -> mux2/40
  MapleSimParameters41/1 -> mux2/41
  MapleSimParameters42/1 -> mux2/42
  MapleSimParameters43/1 -> mux2/43
  MapleSimParameters44/1 -> mux2/44
  MapleSimParameters45/1 -> mux2/45
  MapleSimParameters46/1 -> mux2/46
  MapleSimParameters47/1 -> mux2/47
  MapleSimParameters48/1 -> mux2/48
  MapleSimParameters49/1 -> mux2/49
  MapleSimParameters50/1 -> mux2/50
  MapleSimParameters51/1 -> mux2/51
  MapleSimParameters52/1 -> mux2/52
  MapleSimParameters53/1 -> mux2/53
  MapleSimParameters54/1 -> mux2/54
  MapleSimParameters55/1 -> mux2/55
  MapleSimParameters56/1 -> mux2/56
  MapleSimParameters57/1 -> mux2/57
  MapleSimParameters58/1 -> mux2/58
  MapleSimParameters59/1 -> mux2/59
  MapleSimParameters60/1 -> mux2/60
  MapleSimParameters61/1 -> mux2/61
  MapleSimParameters62/1 -> mux2/62
  MapleSimParameters63/1 -> mux2/63
  MapleSimParameters64/1 -> mux2/64
  MapleSimParameters65/1 -> mux2/65
  MapleSimParameters66/1 -> mux2/66
  MapleSimParameters67/1 -> mux2/67
  mux2/1 -> sfn/2
  mux/1 -> sfn/3
  i_J_Drum/1 -> mux/1
  i_m_unb/1 -> mux/2
  i_temp_rot/1 -> mux/3
  i_temp_stat/1 -> mux/4
  i_va/1 -> mux/5
  i_vb/1 -> mux/6
  i_vc/1 -> mux/7
  sfn/1 -> demux/1
  demux/1 -> o_Ld/1
  demux/2 -> o_Lq/1
  demux/3 -> o_ea/1
  demux/4 -> o_eb/1
  demux/5 -> o_ec/1
  demux/6 -> o_ia/1
  demux/7 -> o_ib/1
  demux/8 -> o_ic/1
  demux/9 -> o_id/1
  demux/10 -> o_iq/1
  demux/11 -> o_omega_e/1
  demux/12 -> o_omega_m/1
  demux/13 -> o_p_rot_loss/1
  demux/14 -> o_p_shaft/1
  demux/15 -> o_pe_abc/1
  demux/16 -> o_pe_b/1
  demux/17 -> o_pe_dq/1
  demux/18 -> o_tau_e/1
  demux/19 -> o_tau_rot_loss/1
  demux/20 -> o_tau_shaft/1
  demux/21 -> o_theta_e/1
  demux/22 -> o_theta_m/1
